simulink model "Fault_Tolerant_Motor_Control"  (R2023b)
settings: Solver=ode23  StartTime=0.0  StopTime=1  RelTol=1e-7
values from neighbouring files (symbols this model uses):
  a = 0.01    [Parameters.m]
  Fc_EMF = 60    [Parameters.m]
  Imax = 95    [Parameters.m]
  J = 0.01    [Parameters.m]
  K_SMO = 20    [Parameters.m]
  Kb_PLL = 50    [Parameters.m]
  Ki_PLL = 9    [Parameters.m]
  Ki_w = 210    [Parameters.m]
  Kp_PLL = 1    [Parameters.m]
  Kp_w = 2.9    [Parameters.m]
  Ld = 0.00047    [Parameters.m]
  Lq = 0.00047    [Parameters.m]
  m = 0.06    [Parameters.m]
  P = 4    [Parameters.m]
  Pmax = 50000    [Parameters.m]
  Psi = 0.1    [Parameters.m]
  Rs = 0.079    [Parameters.m]
  Te_max = 80    [Parameters.m]
  theta_offset = 0    [Parameters.m]
  Ts = 2e-6    (= 2e-06)    [Parameters.m]
  Tsc = 5e-05    [Parameters.m]
  Vdc = 370    [Parameters.m]
undefined symbols (not defined in the file or in its folder): DiscIntNeverNeededParam, ee_sli_rtmsupport, gcbh
libraries: fl_lib x18, nesl_utility x17, ee_lib x11, simulink x6, eeTransforms x2, mcbcontrolslib x2, eePmsmCurrentController x1, eePwmGeneratorTwoLevel x1, slpidlib x1, eeDiscretePi x1, batteryecm_lib x1, eeResolverToDigitalConverter x1
(part 1 of 2)
settings Model: Creator=sm103  LastModifiedBy=sm103
settings DebuggingCC: ParameterPrecisionLossMsg=none  UnderSpecifiedDimensionMsg=warning

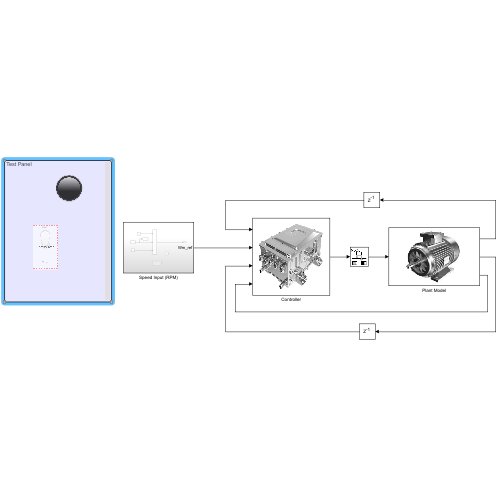
[thumbnail: Simulink's stored preview of the top-level diagram]
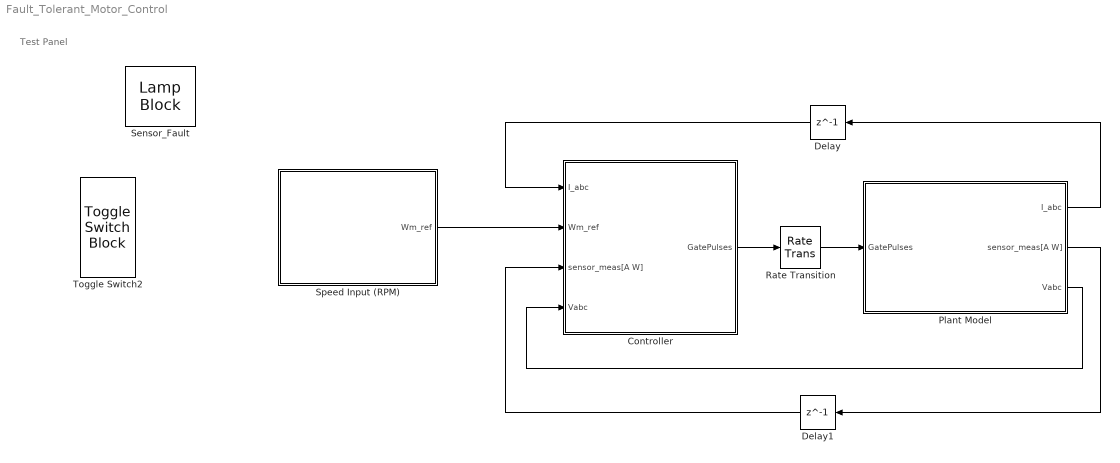
== system Fault_Tolerant_Motor_Control ==
  note: Test Panel
  Controller : Subsystem
      mask Display: image('ev-controller-4.jpeg');
  Delay : Delay  DelayLength=1
  Delay1 : Delay  DelayLength=1
  Plant Model : Subsystem
      mask Display: image('PMSM.jfif');
  Rate Transition : RateTransition  OutPortSampleTime=Ts
  Sensor_Fault : LampBlock  LabelPosition=Hide
  Speed Input (RPM) : Subsystem
  Toggle Switch2 : ToggleSwitchBlock  LabelPosition=Hide
      settings: Values={{'Stop', 'Start'}, [0 1]}
  wires:
  Controller/1(GatePulses) -> Rate Transition/1
  Rate Transition/1 -> Plant Model/1(GatePulses)
  Plant Model/1(I_abc) -> Delay/1
  Delay/1 -> Controller/1(I_abc)
  Plant Model/2(sensor_meas[A W]) -> Delay1/1
  Plant Model/3(Vabc) -> Controller/4(Vabc)
  Delay1/1 -> Controller/3(sensor_meas[A W])
  Speed Input (RPM)/1(Wm_ref) -> Controller/2(Wm_ref)

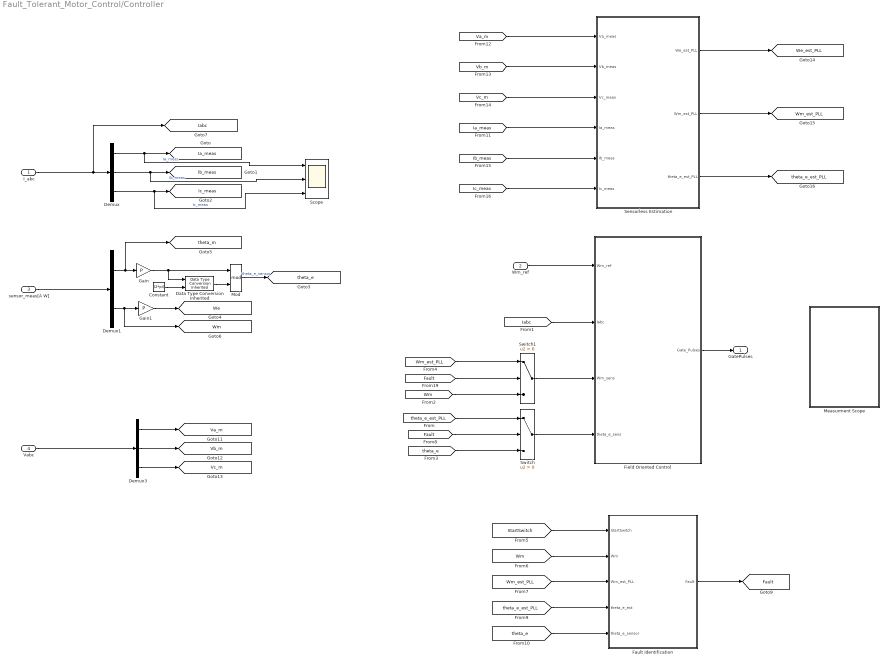
== system Fault_Tolerant_Motor_Control/Controller ==
  I_abc : Inport
  Wm_ref : Inport  Port=2
  sensor_meas[A W] : Inport  Port=3
  Vabc : Inport  Port=4
  Constant : Constant  Value=(2*pi)
  Data Type Conversion Inherited : simulink/Signal Attributes/Data Type Conversion Inherited  ConvertRealWorld=Real World Value  DoSatur=off
  Demux : Demux  Outputs=3
  Demux1 : Demux  Outputs=2
  Demux3 : Demux  Outputs=3
  Fault Identification : Subsystem
  Field Oriented Control : Subsystem
  Gain : Gain  Gain=P
  Gain1 : Gain  Gain=P
  Measurment Scope : Subsystem
  Mod : Math  Operator=mod
  Scope : Scope  NumInputPorts=3
  Sensorless Estimation : Subsystem
  Switch : Switch  Criteria=u2 > Threshold  SaturateOnIntegerOverflow=off  InputSameDT=off
  Switch1 : Switch  Criteria=u2 > Threshold  SaturateOnIntegerOverflow=off  InputSameDT=off
  GatePulses : Outport
  tag scope: Fault=global, Ia_meas=global, Iabc=global, Ib_meas=global, Ic_meas=global, Va_m=global, Vb_m=global, Vc_m=global, We=global, We_est_PLL=global, Wm=global, Wm_est_PLL=global, theta_e=global, theta_e_est_PLL=global, theta_m=global
  wires:
  I_abc/1 -> [Iabc], Demux/1
  Demux/1 -> Scope/1, [Ia_meas]  "Ia_meas"
  Demux/2 -> Scope/2, [Ib_meas]  "Ib_meas"
  Demux/3 -> Scope/3, [Ic_meas]  "Ic_meas"
  sensor_meas[A W]/1 -> Demux1/1
  Demux1/2 -> [Wm], Gain1/1
  Demux1/1 -> [theta_m], Gain/1
  Gain1/1 -> [We]
  Gain/1 -> Data Type Conversion Inherited/1, Mod/1
  Mod/1 -> [theta_e]  "theta_e_sensor"
  Data Type Conversion Inherited/1 -> Mod/2
  Constant/1 -> Data Type Conversion Inherited/2
  Vabc/1 -> Demux3/1
  Demux3/1 -> [Va_m]
  Demux3/2 -> [Vb_m]
  Demux3/3 -> [Vc_m]
  [Iabc] -> Field Oriented Control/2(Iabc)
  Field Oriented Control/1(Gate_Pulses) -> GatePulses/1
  Switch/1 -> Field Oriented Control/4(theta_e_sens)
  [theta_e_est_PLL] -> Switch/1
  Sensorless Estimation/1(We_est_PLL) -> [We_est_PLL]
  Sensorless Estimation/2(Wm_est_PLL) -> [Wm_est_PLL]
  Sensorless Estimation/3("theta_e_est_PLL ") -> [theta_e_est_PLL]
  [Va_m] -> Sensorless Estimation/1(Va_meas)
  [Vb_m] -> Sensorless Estimation/2(Vb_meas)
  [Vc_m] -> Sensorless Estimation/3(Vc_meas)
  Wm_ref/1 -> Field Oriented Control/1(Wm_ref)
  Fault Identification/1(Fault) -> [Fault]
  [StartSwitch] -> Fault Identification/1(StartSwitch)
  [Wm] -> Fault Identification/2(Wm)
  [Wm_est_PLL] -> Fault Identification/3(Wm_est_PLL)
  [theta_e_est_PLL] -> Fault Identification/4(theta_e_est)
  [theta_e] -> Fault Identification/5(theta_e_sensor)
  [Wm_est_PLL] -> Switch1/1
  [Wm] -> Switch1/3
  [Ia_meas] -> Sensorless Estimation/4(Ia_meas)
  [Ib_meas] -> Sensorless Estimation/5(Ib_meas)
  [Ic_meas] -> Sensorless Estimation/6(Ic_meas)
  [theta_e] -> Switch/3
  Switch1/1 -> Field Oriented Control/3(Wm_sens)
  [Fault] -> Switch/2
  [Fault] -> Switch1/2

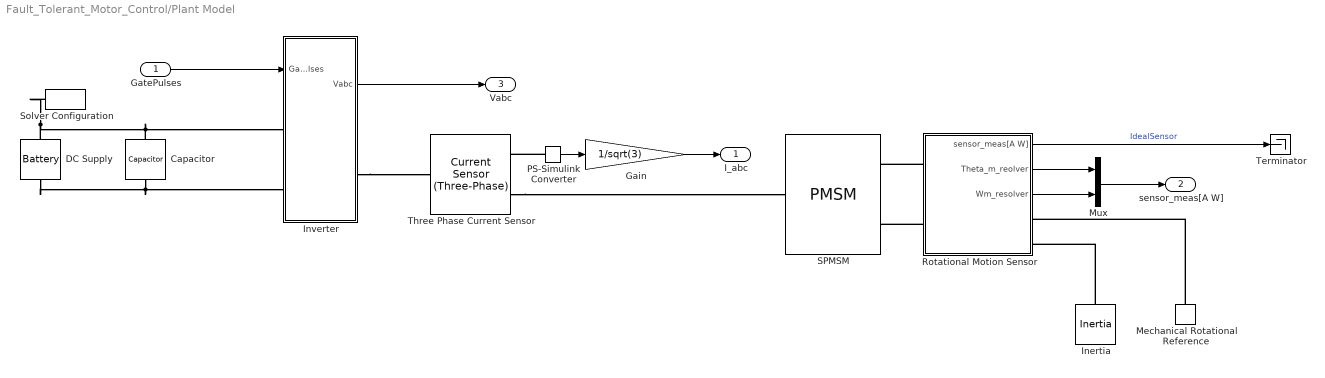
== system Fault_Tolerant_Motor_Control/Plant Model ==
  GatePulses : Inport
  Capacitor : ee_lib/Passive/Capacitor  cap_option=ee.enum.passive.capacitor.capOption.const  c=1e-6 F  Cvec=[1e-05, 1e-06] F  Vvec=[0, 10] V  CV_table_symmetry=ee.enum.passive.capacitor.tableSymmetry.yes  f_vec=[1, 10] kHz  DFext_vec=[.8, 1.2]  enable_C_tol=ee.enum.toleranceApplication.none  averaging_period=0 s  C_tol=5  tol_distribution=ee.enum.toleranceDistribution.uniform  nSigma=4  r=1e-6 Ohm  g=0 1/Ohm  enable_operating_limits=ee.enum.enable.no  operating_limit_action=ee.enum.passive.reportOpLim.warn  max_working_voltage_range=[-25, 25] V  power_rating=1 W  enable_faults=ee.enum.enable.no  fault_action=simscape.enum.assert.action.none  Cscale_faulted=100  R_faulted=1e-3 Ohm  G_faulted=0 1/Ohm  tau_fault=1e-3 s  fault_trigger=ee.enum.faults.faultTrigger.temporal  t_fault=1 s  max_permissible_voltage_range=[-100, 100] V  t_fail_on_voltage=1 s  i_specify=off  i_priority=None  i=0 A  i_nominal_specify=off  i_nominal_unit=A  i_nominal_value=1  v_specify=off  v_priority=None  v=0 V  v_nominal_specify=off  v_nominal_unit=V  v_nominal_value=1  vc_specify=off  vc_priority=High  vc=0 V  vc_nominal_specify=off  vc_nominal_unit=V  vc_nominal_value=1
  DC Supply : batteryecm_lib/Battery  Vnom=Vdc V  prm_dir=simscape.enum.battery.prm_dir.disabled  R1_dis=2 Ohm  R1_ch=2 Ohm  R1=0.01 Ohm  prm_AH=simscape.enum.battery.prm_AH.infinite  AH=50 A*hr  V1=11.5 V  AH1=25 A*hr  prm_R2=simscape.enum.battery.prm_R2.disabled  R2=2000 Ohm  Tmeas=298.15 K  charge_measurement_port=simscape.enum.battery.enable.no  prm_dyn=simscape.enum.battery.prm_dyn.off  Rp1=0.005 Ohm  tau1=30 s  Rp2=0.005 Ohm  tau2=30 s  Rp3=0.005 Ohm  tau3=30 s  Rp4=0.005 Ohm  tau4=30 s  Rp5=0.005 Ohm  tau5=30 s  prm_fade=simscape.enum.battery.prm_fade.disabled  N_fade=100  AH_fade=45 A*hr  R1_fade=2.02 Ohm  R1_ch_fade=2.02 Ohm  V1_fade=10.35 V  prm_age=simscape.enum.battery.prm_age.disabled  prm_age_OCV=simscape.enum.battery.prm_age_OCV.OCV  OCV_age=0.9  SOC_age=60  Tmeas_age=298.15 K  delta_time_age_vec=[0] d  temperature_age_vec=[273] K  OCV_scaling_age=2.2134e6  OCV_offset_age=1.632e6  temp_exp_age=0.515833569 V  t_exp_age=0.75  Vnom_T2=12 V  R1_T2=2.2 Ohm  R1_T2_dis=2.2 Ohm  R1_T2_ch=2.2 Ohm  V1_T2=11.4 V  R2_T2=2200 Ohm  Rp1_T2=0.005 Ohm  tau1_T2=30 s  Rp2_T2=0.005 Ohm  tau2_T2=30 s  Rp3_T2=0.005 Ohm  tau3_T2=30 s  Rp4_T2=0.005 Ohm  tau4_T2=30 s  Rp5_T2=0.005 Ohm  tau5_T2=30 s  Tmeas2=273.15 K  thermal_port=simscape.enum.thermaleffects.omit  thermal_mass=30000 J/K  i_specify=off  i_priority=None  i=0 A  i_nominal_specify=off  i_nominal_unit=A  i_nominal_value=1  v_specify=off  v_priority=None  v=0 V  v_nominal_specify=off  v_nominal_unit=V  v_nominal_value=1  charge_specify=on  charge_priority=High  charge=7000 A*hr  charge_nominal_specify=off  charge_nominal_unit=A*hr  charge_nominal_value=1  num_cycles_specify=off  num_cycles_priority=High  num_cycles=0  num_cycles_nominal_specify=off  num_cycles_nominal_unit=1  num_cycles_nominal_value=1  temperature_specify=off  temperature_priority=High  temperature=298.15 K  temperature_nominal_specify=off  temperature_nominal_unit=K  temperature_nominal_value=1
  Gain : Gain  Gain=1/sqrt(3)
  Inertia : fl_lib/Mechanical/Rotational Elements/Inertia  inertia=J kg*m^2  num_ports=foundation.enum.numPorts2.one  w_specify=on  w_priority=High  w=0 rad/s  w_nominal_specify=off  w_nominal_unit=rad/s  w_nominal_value=0  t_specify=off  t_priority=None  t=0 N*m  t_nominal_specify=off  t_nominal_unit=N*m  t_nominal_value=0
  Inverter : Subsystem
  Mechanical Rotational Reference : fl_lib/Mechanical/Rotational Elements/Mechanical Rotational Reference
  Mux : Mux  Inputs=2
  PS-Simulink Converter : nesl_utility/PS-Simulink Converter  PhysicalDomain=network_engine_domain  SubClassName=ps_output  LeftPortType=input  RightPortType=output  PseudoPeriodic=off  Frequencies=[]  VectorFormat=inherit  Unit=inherit  AffineConversion=off
  Rotational Motion Sensor : Subsystem
  SPMSM : ee_lib/Electromechanical/Permanent Magnet/PMSM  port_option=ee.enum.threePhasePort.composite  winding_type=ee.enum.statorconnection.wye  machine_param=ee.enum.pmsm.parameterization.constant  nPolePairs=P  pmflux_param=ee.enum.pmflux.fluxlinkage  pm_flux_linkage=Psi Wb  torque_constant=0.18 N*m/A  back_emf_constant=0.18 V*s/rad  stator_param=ee.enum.statorparam.LdLqL0  Ld=Ld H  Lq=Lq H  idVec=[-200, 0, 200] A  iqVec=[-200, 0, 200] A  LdMatrix=0.0002 * ones(3, 3) H  LqMatrix=0.0002 * ones(3, 3) H  PmMatrix=0.1 * ones(3, 3) Wb  ktMatrix=0.18 * ones(3, 3) N*m/A  keMatrix=0.18 * ones(3, 3) V*s/rad  L0=0.00016 H  Ls=0.0002 H  Lm=-0.00002 H  Ms=0.00002 H  Rs=Rs Ohm  zero_sequence=ee.enum.park.zerosequence.exclude  axes_param=ee.enum.rotorangle.qaxis  loss_param=ee.enum.ironloss.none  losses_oc=[0, 0, 0] W  losses_sc=[0, 0, 0] W  f_losses=60 Hz  Isc_losses=95 A  J=0.01 kg*m^2  lam=0 N*m*s/rad  i_d_specify=off  i_d_priority=None  i_d=0 A  i_d_nominal_specify=off  i_d_nominal_unit=A  i_d_nominal_value=1  i_q_specify=off  i_q_priority=None  i_q=0 A  i_q_nominal_specify=off  i_q_nominal_unit=A  i_q_nominal_value=1  torque_specify=off  torque_priority=None  torque=0 N*m  torque_nominal_specify=off  torque_nominal_unit=N*m  torque_nominal_value=1  angular_velocity_specify=on  angular_velocity_priority=High  angular_velocity=0 rpm  angular_velocity_nominal_specify=off  angular_velocity_nominal_unit=rpm  angular_velocity_nominal_value=1  angular_position_specify=on  angular_position_priority=High  angular_position=0 deg  angular_position_nominal_specify=off  angular_position_nominal_unit=deg  angular_position_nominal_value=1  alpha=3.93e-3 1/K  alpha_flux=-0.001 1/K  Tmeas=298.15 K  stator_thermal_mass=100 J/K  rotor_thermal_mass=200 J/K  Rm_percent_rotor=90  Rd_percent_rotor=30  temperatureA_specify=off  temperatureA_priority=High  temperatureA=25 degC  temperatureA_nominal_specify=off  temperatureA_nominal_unit=degC  temperatureA_nominal_value=1  temperatureB_specify=off  temperatureB_priority=High  temperatureB=25 degC  temperatureB_nominal_specify=off  temperatureB_nominal_unit=degC  temperatureB_nominal_value=1  temperatureC_specify=off  temperatureC_priority=High  temperatureC=25 degC  temperatureC_nominal_specify=off  temperatureC_nominal_unit=degC  temperatureC_nominal_value=1  temperatureR_specify=off  temperatureR_priority=High  temperatureR=25 degC  temperatureR_nominal_specify=off  temperatureR_nominal_unit=degC  temperatureR_nominal_value=1
      settings: InternalSimscapePortConfiguration="{\"Bottom\":[],\"Left\":[{\"id\":\"N\",\"label\":\"~\",\"type\":\"foundation.electrical.three_phase\"}],\"Right\":[{\"id\":\"R\",\"label\":\"R\",\"type\":\"foundation.mechanical.rotational.rotational\"},{\"id\":\"C\",\"label\":\"C\",\"type\":\"foundation.mechanical.rotational.rotational\"}],\"Top\":[]}"
  Solver Configuration : nesl_utility/Solver Configuration  PhysicalDomain=network_engine_domain  SubClassName=solver  LeftPortType=input  RightPortType=generic  Tones=[]  Harmonics=[]  SimulateNoise=off  Profile=off  UseLocalSampling=off  EnableSwitchedLinearOptims=on  FrequencyDomain=off  UseCCode=off  RelTol=0.001  AbsTol=1e-06  MinStep=1e-09  ToWorkspace=off  RevertToSquareIcSolve=off  NumHomotopyIterations=100  PhasorMode=off  PhasorModeNumHarmonics=1  ConsistencySolver=NEWTON_FTOL  IndexReductionMethod=DerivativeReplacement  DoDC=off  ResidualTolerance=1e-9  ConsistencyTolSource=GLOBAL  ConsistencyAbsTol=0.001  ConsistencyRelTol=0.001  ConsistencyTolFactor=0.001  UseLocalSolver=on  LocalSolverChoice=NE_BACKWARD_EULER_ADVANCER  ResolveIndetEquations=on  FunctionEvalNumThread=1  LocalSolverSampleTime=Ts  DoFixedCost=on  MaxNonlinIter=4  MaxModeIter=2  ComputeImpulses=off  ImpulseIterations=2  LinearAlgebra=auto  LinearAlgebraNumThread=0  EquationFormulation=NE_TIME_EF  DelaysMemoryBudget=1024  AutomaticFiltering=on  FilteringTimeConstant=0.001  PartitionStorageMethod=AS_NEEDED  PartitionMemoryBudget=1024  PartitionMethod=FAST  MultibodyUseLocalSolver=off  MultibodyLocalSolverChoice=ODE1  MultibodyLocalSolverSampleTime=0.001
  Terminator : Terminator
  Three Phase Current Sensor : ee_lib/Sensors & Transducers/Current Sensor (Three-Phase)
  I_abc : Outport
  sensor_meas[A W] : Outport  Port=2
  Vabc : Outport  Port=3
  wires:
  Gain/1 -> I_abc/1
  PS-Simulink Converter/1 -> Gain/1
  Rotational Motion Sensor/1(sensor_meas[A W]) -> Terminator/1  "IdealSensor"
  GatePulses/1 -> Inverter/1(GatePulses)
  Inverter/1(Vabc) -> Vabc/1
  Rotational Motion Sensor/2(Theta_m_reolver) -> Mux/1
  Rotational Motion Sensor/3(Wm_resolver) -> Mux/2
  Mux/1 -> sensor_meas[A W]/1
  connections:
  Three Phase Current Sensor/RConn2 -- SPMSM/LConn1
  Mechanical Rotational Reference/LConn1 -- Rotational Motion Sensor/RConn1
  DC Supply/LConn1 -- Inverter/LConn1 -- Capacitor/LConn1 -- Solver Configuration/RConn1
  Inverter/RConn1 -- Three Phase Current Sensor/LConn1
  PS-Simulink Converter/LConn1 -- Three Phase Current Sensor/RConn1
  Rotational Motion Sensor/LConn1 -- SPMSM/RConn1
  DC Supply/RConn1 -- Capacitor/RConn1 -- Inverter/LConn2
  Rotational Motion Sensor/LConn2 -- SPMSM/RConn2
  Inertia/LConn1 -- Rotational Motion Sensor/RConn2

== system Fault_Tolerant_Motor_Control/Speed Input (RPM) ==
  Constant : Constant  Commented=on  Value=1000
  Constant2 : Constant
  Constant3 : Constant  Value=0
  Signal Editor : SignalEditorBlockLib/Signal Editor  Commented=on  FileName=SpeedProfile1.mat  ActiveScenario=Scenario  ActiveSignal=Signal 1  IsBus=off  OutputBusObjectStr=Bus: BusObject  SampleTime=0  Interpolate=off  ZeroCross=off  OutputAfterFinalValue=Setting to zero  Unit=inherit  PreserveSignalName=on  ApplySigPropsToAllScenarios=on  ApplySigPropsToAllSignals=off
  Step : Step  Time=0.5  Before=1000  After=2000  SampleTime=0
  Switch1 : Switch  Criteria=u2 > Threshold  SaturateOnIntegerOverflow=off  InputSameDT=off
  Wm_ref : Outport
  tag scope: StartSwitch=global
  wires:
  Constant2/1 -> [StartSwitch], Switch1/2
  Constant3/1 -> Switch1/3
  Step/1 -> Switch1/1
  Switch1/1 -> Wm_ref/1

== system Fault_Tolerant_Motor_Control/Controller/Fault Identification ==
  StartSwitch : Inport
  Wm : Inport  Port=2
  Wm_est_PLL : Inport  Port=3
  theta_e_est : Inport  Port=4
  theta_e_sensor : Inport  Port=5
  Chart : Stateflow chart  TreatAsAtomicUnit=on
  Fault : Outport
  wires:
  Wm/1 -> Chart/2(Wm)
  StartSwitch/1 -> Chart/1(StartSwitch)
  Wm_est_PLL/1 -> Chart/3(Wm_est_PLL)
  Chart/1(Fault) -> Fault/1
  theta_e_est/1 -> Chart/4(theta_e_est)
  theta_e_sensor/1 -> Chart/5(theta_e_sensor)

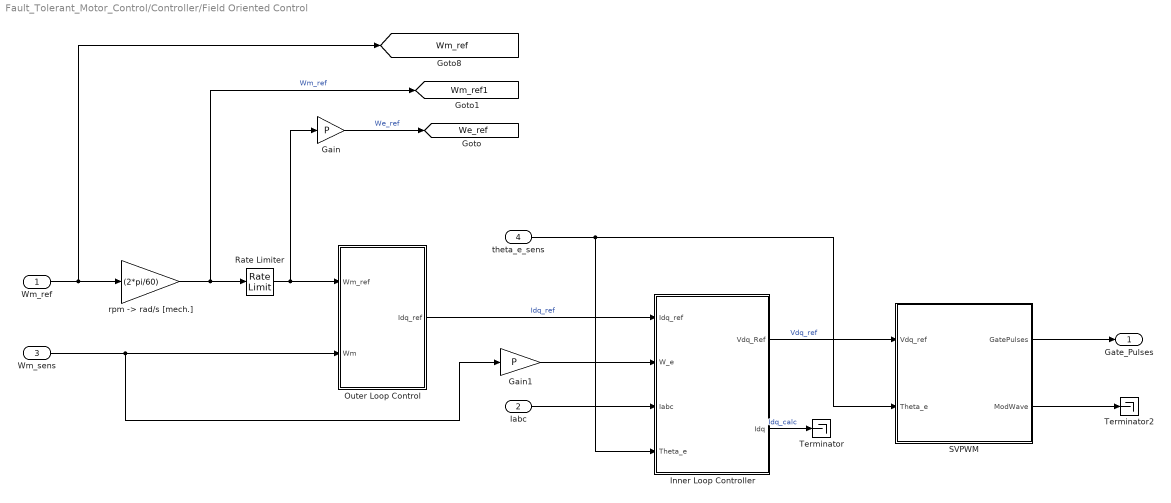
== system Fault_Tolerant_Motor_Control/Controller/Field Oriented Control ==
  Wm_ref : Inport
  Iabc : Inport  Port=2
  Wm_sens : Inport  Port=3
  theta_e_sens : Inport  Port=4
  Gain : Gain  Gain=P
  Gain1 : Gain  Gain=P
  Inner Loop Controller : Subsystem
  Outer Loop Control : Subsystem
  Rate Limiter : RateLimiter  RisingSlewLimit=(Te_max/J)  FallingSlewLimit=-(Te_max/J)  SampleTimeMode=inherited
  SVPWM : Subsystem
  Terminator : Terminator
  Terminator2 : Terminator
  "rpm -> rad/s [mech.]" : Gain  Gain=(2*pi/60)
  Gate_Pulses : Outport
  tag scope: We_ref=global, Wm_ref1=global, Wm_ref=global
  wires:
  Wm_ref/1 -> "rpm -> rad/s [mech.]"/1, [Wm_ref]
  "rpm -> rad/s [mech.]"/1 -> [Wm_ref1], Rate Limiter/1  "Wm_ref"
  Rate Limiter/1 -> Gain/1, Outer Loop Control/1(Wm_ref)
  Iabc/1 -> Inner Loop Controller/3(Iabc)
  Wm_sens/1 -> Outer Loop Control/2(Wm), Gain1/1
  theta_e_sens/1 -> Inner Loop Controller/4(Theta_e), SVPWM/2(Theta_e)
  Gain/1 -> [We_ref]  "We_ref"
  Outer Loop Control/1(Idq_ref) -> Inner Loop Controller/1(Idq_ref)  "Idq_ref"
  Inner Loop Controller/1(Vdq_Ref) -> SVPWM/1(Vdq_ref)  "Vdq_ref"
  Gain1/1 -> Inner Loop Controller/2(W_e)
  SVPWM/1(GatePulses) -> Gate_Pulses/1
  Inner Loop Controller/2(Idq) -> Terminator/1  "Idq_calc"
  SVPWM/2(ModWave) -> Terminator2/1

== system Fault_Tolerant_Motor_Control/Controller/Measurment Scope ==
  Position Error : Subsystem
  Scope : Scope  NumInputPorts=10
  Speed Error : Subsystem
  wires:
  [theta_e] -> Scope/4  "Resolver Electrical Angle (rad)"
  [theta_e_est_PLL] -> Scope/5  "Estimated Electrical Angle (rad)"
  [Wm_est_PLL] -> Scope/2  "Estimated Mechanical Speed (rad/s)"
  [Wm] -> Scope/3  "Resolver Mechanical Speed (rad/s)"
  [Wm_ref1] -> Scope/1  "Mechanical Speed Reference (rad/s)"
  Speed Error/1(Out1) -> Scope/6  "Speed Error (rad/s)"
  Position Error/1(Out1) -> Scope/7  "Position Error (rad)"
  [Fault] -> Scope/8  "Sensor Fault"
  [theta_e_testSensor] -> Scope/9  "Electrical angle test sensor (rad)"
  [Wm_testSensor] -> Scope/10  "Mechanical Speed from test sensor (rad/s)"

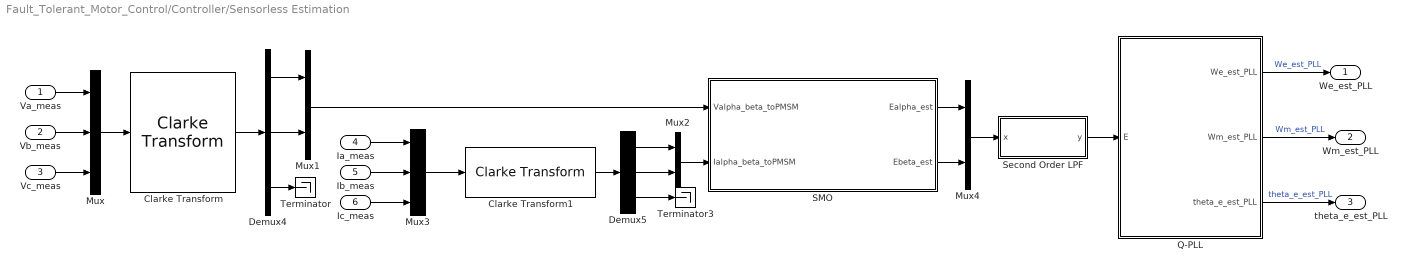
== system Fault_Tolerant_Motor_Control/Controller/Sensorless Estimation ==
  Va_meas : Inport
  Vb_meas : Inport  Port=2
  Vc_meas : Inport  Port=3
  Ia_meas : Inport  Port=4
  Ib_meas : Inport  Port=5
  Ic_meas : Inport  Port=6
  Clarke Transform : mcbcontrolslib/Clarke Transform  VariantControl=Variant2  PhaseInput=Three inputs  EnPowerInv=off
      settings: LibrarySourceBlock=mcbhdllib/Controls/Math Transforms/Clarke Transform
  Clarke Transform1 : mcbcontrolslib/Clarke Transform  VariantControl=Variant2  PhaseInput=Three inputs  EnPowerInv=off
      settings: LibrarySourceBlock=mcbhdllib/Controls/Math Transforms/Clarke Transform
  Demux4 : Demux  Outputs=3
  Demux5 : Demux  Outputs=3
  Mux : Mux  Inputs=3
  Mux1 : Mux  Inputs=2
  Mux2 : Mux  Inputs=2
  Mux3 : Mux  Inputs=3
  Mux4 : Mux  Inputs=2
  Q-PLL : Subsystem
  SMO : Subsystem
  Second Order LPF : Subsystem
  Terminator : Terminator
  Terminator3 : Terminator
  We_est_PLL : Outport
  Wm_est_PLL : Outport  Port=2
  "theta_e_est_PLL " : Outport  Port=3
  wires:
  Demux4/2 -> Mux1/2
  Q-PLL/2(Wm_est_PLL) -> Wm_est_PLL/1  "Wm_est_PLL"
  Demux5/3 -> Terminator3/1
  Mux2/1 -> SMO/2(Ialpha_beta_toPMSM)
  Mux3/1 -> Clarke Transform1/1
  Demux5/2 -> Mux2/2
  Demux5/1 -> Mux2/1
  Va_meas/1 -> Mux/1
  Mux/1 -> Clarke Transform/1
  Vb_meas/1 -> Mux/2
  Demux4/3 -> Terminator/1
  Clarke Transform/1 -> Demux4/1
  Q-PLL/1(We_est_PLL) -> We_est_PLL/1  "We_est_PLL"
  Ic_meas/1 -> Mux3/3
  Ia_meas/1 -> Mux3/1
  Mux1/1 -> SMO/1(Valpha_beta_toPMSM)
  Clarke Transform1/1 -> Demux5/1
  Ib_meas/1 -> Mux3/2
  Vc_meas/1 -> Mux/3
  Demux4/1 -> Mux1/1
  Q-PLL/3(theta_e_est_PLL) -> "theta_e_est_PLL "/1  "theta_e_est_PLL"
  SMO/1(Ealpha_est) -> Mux4/1
  SMO/2(Ebeta_est) -> Mux4/2
  Second Order LPF/1(y) -> Q-PLL/1(E)
  Mux4/1 -> Second Order LPF/1(x)

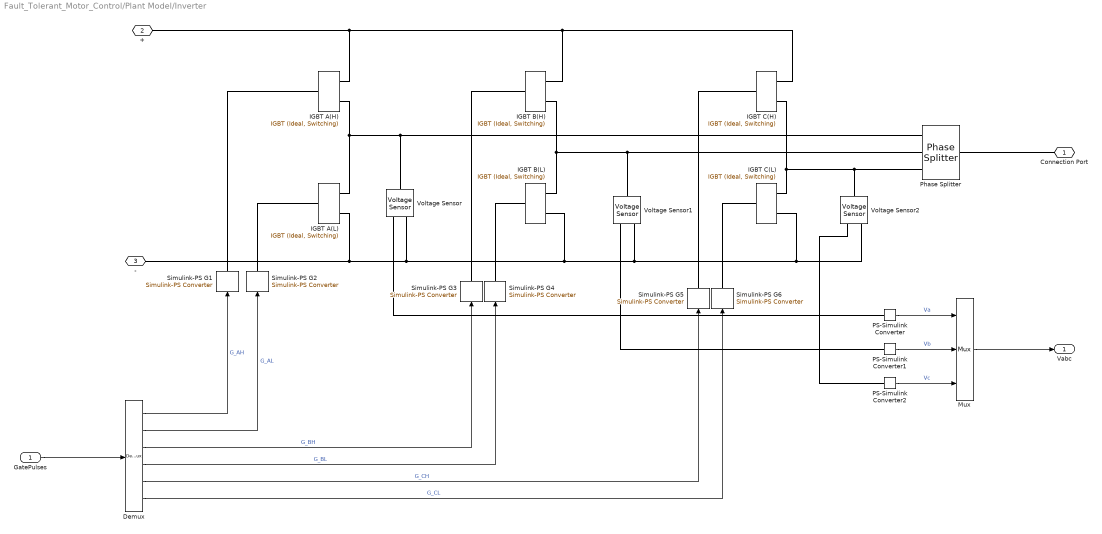
== system Fault_Tolerant_Motor_Control/Plant Model/Inverter ==
  GatePulses : Inport
  Demux : Demux  Outputs=6
  IGBT A(H) : ee_lib/Semiconductors & Converters/IGBT (Ideal, Switching)  port_option=ee.enum.controlport.ps  Vf=0.8 V  Ron=0.001 Ohm  Goff=1e-5 S  Vth=0.5 V  diode_param=ee.enum.converters.protectiondiode.nodynamics  diode_Vf=0.8 V  diode_Ron=0.001 Ohm  diode_Goff=1e-5 S  diode_C=5e-8 F  diode_iRM=-235 A  diode_iF=300 A  diode_idot=-50 A/us  diode_trr_param=1  diode_trr_factor=3  diode_trr=15 us  diode_Qrr=1.5e+3 s*uA  ice_specify=off  ice_priority=None  ice=0 A  ice_nominal_specify=off  ice_nominal_unit=A  ice_nominal_value=1  vce_specify=off  vce_priority=None  vce=0 V  vce_nominal_specify=off  vce_nominal_unit=V  vce_nominal_value=1  vge_specify=off  vge_priority=None  vge=0 V  vge_nominal_specify=off  vge_nominal_unit=V  vge_nominal_value=1  thermal_loss_option=ee.enum.converters.thermalLossOption.constantvalues  Von_data=[0, .1, .6, .8, 1, 1.3, 1.6, 2, 2.4; 0, .1, .7, 1, 1.2, 1.5, 1.9, 2.4, 2.8] V  Tj=[298.15, 398.15] K  Iout_data=[0, .1, 1, 5, 10, 20, 40, 70, 100] A  Eon_data=[0, .0024, .024, .12, .2, .48, 1.04, 2.16, 3.24; 0, .003, .03, .15, .25, .6, 1.3, 2.7, 4.05] * 1e-3 J  Eoff_data=[0, .0007, .0066, .033, .066, .17, .33, .83, 1.5; 0, .001, .01, .05, .1, .25, .5, 1.2, 2.2] * 1e-3 J  Eon_data_3D=[zeros(2, 9, 3)] J  Eoff_data_3D=[zeros(2, 9, 3)] J  Tj_loss=[298.15, 398.15] K  Iout_data_loss=[0, .1, 1, 5, 10, 20, 40, 70, 100] A  tabulateWithVce=false  Vce_loss=[0, 150, 300] V  Eon_scalar=22.86e-3 J  Eoff_scalar=17.14e-3 J  Voff=300 V  Iout_scalar=600 A  useCurrentFromPreviousCycle=false  useVoltageFromPreviousCycle=false  diodeModelType=ee.enum.converters.diodeModelType.pwl  diodeTableType=ee.enum.diode.tableType.IfMat  diode_IfMat=[.07, .12, .19, 1.75, 4.24, 7.32, 11.2; .16, .3, .72, 2.14, 4.02, 6.35, 9.12] A  diode_VfMat=[.9, 1.15, 1.25, 1.5, 1.75, 2.17, 2.6, 2.85; .58, .68, .75, 1.1, 1.38, 1.77, 2.27, 2.7] V  diode_TjVec=[25, 125] degC  diode_VfVec=[.5, .7, .9, 1.3, 1.7, 2.1, 2.5] V  diode_IfVec=[.1, .2, .5, 1, 2, 4, 7, 10] A  diode_Vr=-600 V  diode_Ls=150 nH  diode_Erec=0.03 J  diode_rec_loss_model=ee.enum.diode.reverseRecoveryModel.fixed  diode_ErecVal=0 J  diode_scaleWithIandV=true  diode_ErecMat=zeros(2, 3) J  diode_TjrecVec=[298.15, 398.15] K  diode_IfrecVec=[.1, 1, 10] A  diode_IrecVal=10 A  diode_VrecVal=10 V  diode_tFilter=1 / 1000 / 100 s  thermal_network_parameterization=ee.enum.thermalNetworkTopology.external  Rth=[.08, .5] K/W  Rth_Cauer=[.08, .1, .5] K/W  Rth_Foster=[.08, .14, .22, .16] K/W  thermal_mass_parameterization=ee.enum.thermalNetwork.timeconstant  thermal_mass=[.01, .5] J/K  thermal_mass_Cauer=[.01, .1, .5] J/K  thermal_mass_Foster=[.001, .005, .05, .5] J/K  thermal_time_constant=[.001, .2] s  thermal_time_constant_Cauer=[.001, .1, .2] s  thermal_time_constant_Foster=[7e-05, .0007, .01, .08] s  thermal_mass_initial_temperatures=[25, 25] degC  thermal_mass_initial_temperatures_Cauer=[25, 25, 25] degC  junction_thermal_mass=0.01 J/K  Tvec_initial_Foster=[25, 25, 25, 25] degC  no_thermal_network=0  junction_temperature_specify=off  junction_temperature_priority=None  junction_temperature=25 degC  junction_temperature_nominal_specify=off  junction_temperature_nominal_unit=degC  junction_temperature_nominal_value=1  Qj_specify=off  Qj_priority=None  Qj=0 W  Qj_nominal_specify=off  Qj_nominal_unit=W  Qj_nominal_value=1  accumulatedSwitchingLosses_specify=off  accumulatedSwitchingLosses_priority=None  accumulatedSwitchingLosses=0 J
  IGBT A(L) : ee_lib/Semiconductors & Converters/IGBT (Ideal, Switching)  port_option=ee.enum.controlport.ps  Vf=0.8 V  Ron=0.001 Ohm  Goff=1e-5 S  Vth=0.5 V  diode_param=2  diode_Vf=0.8 V  diode_Ron=0.001 Ohm  diode_Goff=1e-5 S  diode_C=5e-8 F  diode_iRM=-235 A  diode_iF=300 A  diode_idot=-50 A/us  diode_trr_param=1  diode_trr_factor=3  diode_trr=15 us  diode_Qrr=1.5e+3 s*uA  ice_specify=off  ice_priority=None  ice=0 A  ice_nominal_specify=off  ice_nominal_unit=A  ice_nominal_value=1  vce_specify=off  vce_priority=None  vce=0 V  vce_nominal_specify=off  vce_nominal_unit=V  vce_nominal_value=1  vge_specify=off  vge_priority=None  vge=0 V  vge_nominal_specify=off  vge_nominal_unit=V  vge_nominal_value=1  thermal_loss_option=ee.enum.converters.thermalLossOption.constantvalues  Von_data=[0, .1, .6, .8, 1, 1.3, 1.6, 2, 2.4; 0, .1, .7, 1, 1.2, 1.5, 1.9, 2.4, 2.8] V  Tj=[298.15, 398.15] K  Iout_data=[0, .1, 1, 5, 10, 20, 40, 70, 100] A  Eon_data=[0, .0024, .024, .12, .2, .48, 1.04, 2.16, 3.24; 0, .003, .03, .15, .25, .6, 1.3, 2.7, 4.05] * 1e-3 J  Eoff_data=[0, .0007, .0066, .033, .066, .17, .33, .83, 1.5; 0, .001, .01, .05, .1, .25, .5, 1.2, 2.2] * 1e-3 J  Eon_data_3D=[zeros(2, 9, 3)] J  Eoff_data_3D=[zeros(2, 9, 3)] J  Tj_loss=[298.15, 398.15] K  Iout_data_loss=[0, .1, 1, 5, 10, 20, 40, 70, 100] A  tabulateWithVce=false  Vce_loss=[0, 150, 300] V  Eon_scalar=22.86e-3 J  Eoff_scalar=17.14e-3 J  Voff=300 V  Iout_scalar=600 A  useCurrentFromPreviousCycle=false  useVoltageFromPreviousCycle=false  diodeModelType=ee.enum.converters.diodeModelType.pwl  diodeTableType=ee.enum.diode.tableType.IfMat  diode_IfMat=[.07, .12, .19, 1.75, 4.24, 7.32, 11.2; .16, .3, .72, 2.14, 4.02, 6.35, 9.12] A  diode_VfMat=[.9, 1.15, 1.25, 1.5, 1.75, 2.17, 2.6, 2.85; .58, .68, .75, 1.1, 1.38, 1.77, 2.27, 2.7] V  diode_TjVec=[25, 125] degC  diode_VfVec=[.5, .7, .9, 1.3, 1.7, 2.1, 2.5] V  diode_IfVec=[.1, .2, .5, 1, 2, 4, 7, 10] A  diode_Vr=-600 V  diode_Ls=150 nH  diode_Erec=0.03 J  diode_rec_loss_model=ee.enum.diode.reverseRecoveryModel.fixed  diode_ErecVal=0 J  diode_scaleWithIandV=true  diode_ErecMat=zeros(2, 3) J  diode_TjrecVec=[298.15, 398.15] K  diode_IfrecVec=[.1, 1, 10] A  diode_IrecVal=10 A  diode_VrecVal=10 V  diode_tFilter=1 / 1000 / 100 s  thermal_network_parameterization=ee.enum.thermalNetworkTopology.external  Rth=[.08, .5] K/W  Rth_Cauer=[.08, .1, .5] K/W  Rth_Foster=[.08, .14, .22, .16] K/W  thermal_mass_parameterization=ee.enum.thermalNetwork.timeconstant  thermal_mass=[.01, .5] J/K  thermal_mass_Cauer=[.01, .1, .5] J/K  thermal_mass_Foster=[.001, .005, .05, .5] J/K  thermal_time_constant=[.001, .2] s  thermal_time_constant_Cauer=[.001, .1, .2] s  thermal_time_constant_Foster=[7e-05, .0007, .01, .08] s  thermal_mass_initial_temperatures=[25, 25] degC  thermal_mass_initial_temperatures_Cauer=[25, 25, 25] degC  junction_thermal_mass=0.01 J/K  Tvec_initial_Foster=[25, 25, 25, 25] degC  no_thermal_network=0  junction_temperature_specify=off  junction_temperature_priority=None  junction_temperature=25 degC  junction_temperature_nominal_specify=off  junction_temperature_nominal_unit=degC  junction_temperature_nominal_value=1  Qj_specify=off  Qj_priority=None  Qj=0 W  Qj_nominal_specify=off  Qj_nominal_unit=W  Qj_nominal_value=1  accumulatedSwitchingLosses_specify=off  accumulatedSwitchingLosses_priority=None  accumulatedSwitchingLosses=0 J
  IGBT B(H) : ee_lib/Semiconductors & Converters/IGBT (Ideal, Switching)  port_option=ee.enum.controlport.ps  Vf=0.8 V  Ron=0.001 Ohm  Goff=1e-5 S  Vth=0.5 V  diode_param=2  diode_Vf=0.8 V  diode_Ron=0.001 Ohm  diode_Goff=1e-5 S  diode_C=5e-8 F  diode_iRM=-235 A  diode_iF=300 A  diode_idot=-50 A/us  diode_trr_param=1  diode_trr_factor=3  diode_trr=15 us  diode_Qrr=1.5e+3 s*uA  ice_specify=off  ice_priority=None  ice=0 A  ice_nominal_specify=off  ice_nominal_unit=A  ice_nominal_value=1  vce_specify=off  vce_priority=None  vce=0 V  vce_nominal_specify=off  vce_nominal_unit=V  vce_nominal_value=1  vge_specify=off  vge_priority=None  vge=0 V  vge_nominal_specify=off  vge_nominal_unit=V  vge_nominal_value=1  thermal_loss_option=ee.enum.converters.thermalLossOption.constantvalues  Von_data=[0, .1, .6, .8, 1, 1.3, 1.6, 2, 2.4; 0, .1, .7, 1, 1.2, 1.5, 1.9, 2.4, 2.8] V  Tj=[298.15, 398.15] K  Iout_data=[0, .1, 1, 5, 10, 20, 40, 70, 100] A  Eon_data=[0, .0024, .024, .12, .2, .48, 1.04, 2.16, 3.24; 0, .003, .03, .15, .25, .6, 1.3, 2.7, 4.05] * 1e-3 J  Eoff_data=[0, .0007, .0066, .033, .066, .17, .33, .83, 1.5; 0, .001, .01, .05, .1, .25, .5, 1.2, 2.2] * 1e-3 J  Eon_data_3D=[zeros(2, 9, 3)] J  Eoff_data_3D=[zeros(2, 9, 3)] J  Tj_loss=[298.15, 398.15] K  Iout_data_loss=[0, .1, 1, 5, 10, 20, 40, 70, 100] A  tabulateWithVce=false  Vce_loss=[0, 150, 300] V  Eon_scalar=22.86e-3 J  Eoff_scalar=17.14e-3 J  Voff=300 V  Iout_scalar=600 A  useCurrentFromPreviousCycle=false  useVoltageFromPreviousCycle=false  diodeModelType=ee.enum.converters.diodeModelType.pwl  diodeTableType=ee.enum.diode.tableType.IfMat  diode_IfMat=[.07, .12, .19, 1.75, 4.24, 7.32, 11.2; .16, .3, .72, 2.14, 4.02, 6.35, 9.12] A  diode_VfMat=[.9, 1.15, 1.25, 1.5, 1.75, 2.17, 2.6, 2.85; .58, .68, .75, 1.1, 1.38, 1.77, 2.27, 2.7] V  diode_TjVec=[25, 125] degC  diode_VfVec=[.5, .7, .9, 1.3, 1.7, 2.1, 2.5] V  diode_IfVec=[.1, .2, .5, 1, 2, 4, 7, 10] A  diode_Vr=-600 V  diode_Ls=150 nH  diode_Erec=0.03 J  diode_rec_loss_model=ee.enum.diode.reverseRecoveryModel.fixed  diode_ErecVal=0 J  diode_scaleWithIandV=true  diode_ErecMat=zeros(2, 3) J  diode_TjrecVec=[298.15, 398.15] K  diode_IfrecVec=[.1, 1, 10] A  diode_IrecVal=10 A  diode_VrecVal=10 V  diode_tFilter=1 / 1000 / 100 s  thermal_network_parameterization=ee.enum.thermalNetworkTopology.external  Rth=[.08, .5] K/W  Rth_Cauer=[.08, .1, .5] K/W  Rth_Foster=[.08, .14, .22, .16] K/W  thermal_mass_parameterization=ee.enum.thermalNetwork.timeconstant  thermal_mass=[.01, .5] J/K  thermal_mass_Cauer=[.01, .1, .5] J/K  thermal_mass_Foster=[.001, .005, .05, .5] J/K  thermal_time_constant=[.001, .2] s  thermal_time_constant_Cauer=[.001, .1, .2] s  thermal_time_constant_Foster=[7e-05, .0007, .01, .08] s  thermal_mass_initial_temperatures=[25, 25] degC  thermal_mass_initial_temperatures_Cauer=[25, 25, 25] degC  junction_thermal_mass=0.01 J/K  Tvec_initial_Foster=[25, 25, 25, 25] degC  no_thermal_network=0  junction_temperature_specify=off  junction_temperature_priority=None  junction_temperature=25 degC  junction_temperature_nominal_specify=off  junction_temperature_nominal_unit=degC  junction_temperature_nominal_value=1  Qj_specify=off  Qj_priority=None  Qj=0 W  Qj_nominal_specify=off  Qj_nominal_unit=W  Qj_nominal_value=1  accumulatedSwitchingLosses_specify=off  accumulatedSwitchingLosses_priority=None  accumulatedSwitchingLosses=0 J
  IGBT B(L) : ee_lib/Semiconductors & Converters/IGBT (Ideal, Switching)  port_option=ee.enum.controlport.ps  Vf=0.8 V  Ron=0.001 Ohm  Goff=1e-5 S  Vth=0.5 V  diode_param=2  diode_Vf=0.8 V  diode_Ron=0.001 Ohm  diode_Goff=1e-5 S  diode_C=5e-8 F  diode_iRM=-235 A  diode_iF=300 A  diode_idot=-50 A/us  diode_trr_param=1  diode_trr_factor=3  diode_trr=15 us  diode_Qrr=1.5e+3 s*uA  ice_specify=off  ice_priority=None  ice=0 A  ice_nominal_specify=off  ice_nominal_unit=A  ice_nominal_value=1  vce_specify=off  vce_priority=None  vce=0 V  vce_nominal_specify=off  vce_nominal_unit=V  vce_nominal_value=1  vge_specify=off  vge_priority=None  vge=0 V  vge_nominal_specify=off  vge_nominal_unit=V  vge_nominal_value=1  thermal_loss_option=ee.enum.converters.thermalLossOption.constantvalues  Von_data=[0, .1, .6, .8, 1, 1.3, 1.6, 2, 2.4; 0, .1, .7, 1, 1.2, 1.5, 1.9, 2.4, 2.8] V  Tj=[298.15, 398.15] K  Iout_data=[0, .1, 1, 5, 10, 20, 40, 70, 100] A  Eon_data=[0, .0024, .024, .12, .2, .48, 1.04, 2.16, 3.24; 0, .003, .03, .15, .25, .6, 1.3, 2.7, 4.05] * 1e-3 J  Eoff_data=[0, .0007, .0066, .033, .066, .17, .33, .83, 1.5; 0, .001, .01, .05, .1, .25, .5, 1.2, 2.2] * 1e-3 J  Eon_data_3D=[zeros(2, 9, 3)] J  Eoff_data_3D=[zeros(2, 9, 3)] J  Tj_loss=[298.15, 398.15] K  Iout_data_loss=[0, .1, 1, 5, 10, 20, 40, 70, 100] A  tabulateWithVce=false  Vce_loss=[0, 150, 300] V  Eon_scalar=22.86e-3 J  Eoff_scalar=17.14e-3 J  Voff=300 V  Iout_scalar=600 A  useCurrentFromPreviousCycle=false  useVoltageFromPreviousCycle=false  diodeModelType=ee.enum.converters.diodeModelType.pwl  diodeTableType=ee.enum.diode.tableType.IfMat  diode_IfMat=[.07, .12, .19, 1.75, 4.24, 7.32, 11.2; .16, .3, .72, 2.14, 4.02, 6.35, 9.12] A  diode_VfMat=[.9, 1.15, 1.25, 1.5, 1.75, 2.17, 2.6, 2.85; .58, .68, .75, 1.1, 1.38, 1.77, 2.27, 2.7] V  diode_TjVec=[25, 125] degC  diode_VfVec=[.5, .7, .9, 1.3, 1.7, 2.1, 2.5] V  diode_IfVec=[.1, .2, .5, 1, 2, 4, 7, 10] A  diode_Vr=-600 V  diode_Ls=150 nH  diode_Erec=0.03 J  diode_rec_loss_model=ee.enum.diode.reverseRecoveryModel.fixed  diode_ErecVal=0 J  diode_scaleWithIandV=true  diode_ErecMat=zeros(2, 3) J  diode_TjrecVec=[298.15, 398.15] K  diode_IfrecVec=[.1, 1, 10] A  diode_IrecVal=10 A  diode_VrecVal=10 V  diode_tFilter=1 / 1000 / 100 s  thermal_network_parameterization=ee.enum.thermalNetworkTopology.external  Rth=[.08, .5] K/W  Rth_Cauer=[.08, .1, .5] K/W  Rth_Foster=[.08, .14, .22, .16] K/W  thermal_mass_parameterization=ee.enum.thermalNetwork.timeconstant  thermal_mass=[.01, .5] J/K  thermal_mass_Cauer=[.01, .1, .5] J/K  thermal_mass_Foster=[.001, .005, .05, .5] J/K  thermal_time_constant=[.001, .2] s  thermal_time_constant_Cauer=[.001, .1, .2] s  thermal_time_constant_Foster=[7e-05, .0007, .01, .08] s  thermal_mass_initial_temperatures=[25, 25] degC  thermal_mass_initial_temperatures_Cauer=[25, 25, 25] degC  junction_thermal_mass=0.01 J/K  Tvec_initial_Foster=[25, 25, 25, 25] degC  no_thermal_network=0  junction_temperature_specify=off  junction_temperature_priority=None  junction_temperature=25 degC  junction_temperature_nominal_specify=off  junction_temperature_nominal_unit=degC  junction_temperature_nominal_value=1  Qj_specify=off  Qj_priority=None  Qj=0 W  Qj_nominal_specify=off  Qj_nominal_unit=W  Qj_nominal_value=1  accumulatedSwitchingLosses_specify=off  accumulatedSwitchingLosses_priority=None  accumulatedSwitchingLosses=0 J
  IGBT C(H) : ee_lib/Semiconductors & Converters/IGBT (Ideal, Switching)  port_option=ee.enum.controlport.ps  Vf=0.8 V  Ron=0.001 Ohm  Goff=1e-5 S  Vth=0.5 V  diode_param=2  diode_Vf=0.8 V  diode_Ron=0.001 Ohm  diode_Goff=1e-5 S  diode_C=5e-8 F  diode_iRM=-235 A  diode_iF=300 A  diode_idot=-50 A/us  diode_trr_param=1  diode_trr_factor=3  diode_trr=15 us  diode_Qrr=1.5e+3 s*uA  ice_specify=off  ice_priority=None  ice=0 A  ice_nominal_specify=off  ice_nominal_unit=A  ice_nominal_value=1  vce_specify=off  vce_priority=None  vce=0 V  vce_nominal_specify=off  vce_nominal_unit=V  vce_nominal_value=1  vge_specify=off  vge_priority=None  vge=0 V  vge_nominal_specify=off  vge_nominal_unit=V  vge_nominal_value=1  thermal_loss_option=ee.enum.converters.thermalLossOption.constantvalues  Von_data=[0, .1, .6, .8, 1, 1.3, 1.6, 2, 2.4; 0, .1, .7, 1, 1.2, 1.5, 1.9, 2.4, 2.8] V  Tj=[298.15, 398.15] K  Iout_data=[0, .1, 1, 5, 10, 20, 40, 70, 100] A  Eon_data=[0, .0024, .024, .12, .2, .48, 1.04, 2.16, 3.24; 0, .003, .03, .15, .25, .6, 1.3, 2.7, 4.05] * 1e-3 J  Eoff_data=[0, .0007, .0066, .033, .066, .17, .33, .83, 1.5; 0, .001, .01, .05, .1, .25, .5, 1.2, 2.2] * 1e-3 J  Eon_data_3D=[zeros(2, 9, 3)] J  Eoff_data_3D=[zeros(2, 9, 3)] J  Tj_loss=[298.15, 398.15] K  Iout_data_loss=[0, .1, 1, 5, 10, 20, 40, 70, 100] A  tabulateWithVce=false  Vce_loss=[0, 150, 300] V  Eon_scalar=22.86e-3 J  Eoff_scalar=17.14e-3 J  Voff=300 V  Iout_scalar=600 A  useCurrentFromPreviousCycle=false  useVoltageFromPreviousCycle=false  diodeModelType=ee.enum.converters.diodeModelType.pwl  diodeTableType=ee.enum.diode.tableType.IfMat  diode_IfMat=[.07, .12, .19, 1.75, 4.24, 7.32, 11.2; .16, .3, .72, 2.14, 4.02, 6.35, 9.12] A  diode_VfMat=[.9, 1.15, 1.25, 1.5, 1.75, 2.17, 2.6, 2.85; .58, .68, .75, 1.1, 1.38, 1.77, 2.27, 2.7] V  diode_TjVec=[25, 125] degC  diode_VfVec=[.5, .7, .9, 1.3, 1.7, 2.1, 2.5] V  diode_IfVec=[.1, .2, .5, 1, 2, 4, 7, 10] A  diode_Vr=-600 V  diode_Ls=150 nH  diode_Erec=0.03 J  diode_rec_loss_model=ee.enum.diode.reverseRecoveryModel.fixed  diode_ErecVal=0 J  diode_scaleWithIandV=true  diode_ErecMat=zeros(2, 3) J  diode_TjrecVec=[298.15, 398.15] K  diode_IfrecVec=[.1, 1, 10] A  diode_IrecVal=10 A  diode_VrecVal=10 V  diode_tFilter=1 / 1000 / 100 s  thermal_network_parameterization=ee.enum.thermalNetworkTopology.external  Rth=[.08, .5] K/W  Rth_Cauer=[.08, .1, .5] K/W  Rth_Foster=[.08, .14, .22, .16] K/W  thermal_mass_parameterization=ee.enum.thermalNetwork.timeconstant  thermal_mass=[.01, .5] J/K  thermal_mass_Cauer=[.01, .1, .5] J/K  thermal_mass_Foster=[.001, .005, .05, .5] J/K  thermal_time_constant=[.001, .2] s  thermal_time_constant_Cauer=[.001, .1, .2] s  thermal_time_constant_Foster=[7e-05, .0007, .01, .08] s  thermal_mass_initial_temperatures=[25, 25] degC  thermal_mass_initial_temperatures_Cauer=[25, 25, 25] degC  junction_thermal_mass=0.01 J/K  Tvec_initial_Foster=[25, 25, 25, 25] degC  no_thermal_network=0  junction_temperature_specify=off  junction_temperature_priority=None  junction_temperature=25 degC  junction_temperature_nominal_specify=off  junction_temperature_nominal_unit=degC  junction_temperature_nominal_value=1  Qj_specify=off  Qj_priority=None  Qj=0 W  Qj_nominal_specify=off  Qj_nominal_unit=W  Qj_nominal_value=1  accumulatedSwitchingLosses_specify=off  accumulatedSwitchingLosses_priority=None  accumulatedSwitchingLosses=0 J
  IGBT C(L) : ee_lib/Semiconductors & Converters/IGBT (Ideal, Switching)  port_option=ee.enum.controlport.ps  Vf=0.8 V  Ron=0.001 Ohm  Goff=1e-5 S  Vth=0.5 V  diode_param=2  diode_Vf=0.8 V  diode_Ron=0.001 Ohm  diode_Goff=1e-5 S  diode_C=5e-8 F  diode_iRM=-235 A  diode_iF=300 A  diode_idot=-50 A/us  diode_trr_param=1  diode_trr_factor=3  diode_trr=15 us  diode_Qrr=1.5e+3 s*uA  ice_specify=off  ice_priority=None  ice=0 A  ice_nominal_specify=off  ice_nominal_unit=A  ice_nominal_value=1  vce_specify=off  vce_priority=None  vce=0 V  vce_nominal_specify=off  vce_nominal_unit=V  vce_nominal_value=1  vge_specify=off  vge_priority=None  vge=0 V  vge_nominal_specify=off  vge_nominal_unit=V  vge_nominal_value=1  thermal_loss_option=ee.enum.converters.thermalLossOption.constantvalues  Von_data=[0, .1, .6, .8, 1, 1.3, 1.6, 2, 2.4; 0, .1, .7, 1, 1.2, 1.5, 1.9, 2.4, 2.8] V  Tj=[298.15, 398.15] K  Iout_data=[0, .1, 1, 5, 10, 20, 40, 70, 100] A  Eon_data=[0, .0024, .024, .12, .2, .48, 1.04, 2.16, 3.24; 0, .003, .03, .15, .25, .6, 1.3, 2.7, 4.05] * 1e-3 J  Eoff_data=[0, .0007, .0066, .033, .066, .17, .33, .83, 1.5; 0, .001, .01, .05, .1, .25, .5, 1.2, 2.2] * 1e-3 J  Eon_data_3D=[zeros(2, 9, 3)] J  Eoff_data_3D=[zeros(2, 9, 3)] J  Tj_loss=[298.15, 398.15] K  Iout_data_loss=[0, .1, 1, 5, 10, 20, 40, 70, 100] A  tabulateWithVce=false  Vce_loss=[0, 150, 300] V  Eon_scalar=22.86e-3 J  Eoff_scalar=17.14e-3 J  Voff=300 V  Iout_scalar=600 A  useCurrentFromPreviousCycle=false  useVoltageFromPreviousCycle=false  diodeModelType=ee.enum.converters.diodeModelType.pwl  diodeTableType=ee.enum.diode.tableType.IfMat  diode_IfMat=[.07, .12, .19, 1.75, 4.24, 7.32, 11.2; .16, .3, .72, 2.14, 4.02, 6.35, 9.12] A  diode_VfMat=[.9, 1.15, 1.25, 1.5, 1.75, 2.17, 2.6, 2.85; .58, .68, .75, 1.1, 1.38, 1.77, 2.27, 2.7] V  diode_TjVec=[25, 125] degC  diode_VfVec=[.5, .7, .9, 1.3, 1.7, 2.1, 2.5] V  diode_IfVec=[.1, .2, .5, 1, 2, 4, 7, 10] A  diode_Vr=-600 V  diode_Ls=150 nH  diode_Erec=0.03 J  diode_rec_loss_model=ee.enum.diode.reverseRecoveryModel.fixed  diode_ErecVal=0 J  diode_scaleWithIandV=true  diode_ErecMat=zeros(2, 3) J  diode_TjrecVec=[298.15, 398.15] K  diode_IfrecVec=[.1, 1, 10] A  diode_IrecVal=10 A  diode_VrecVal=10 V  diode_tFilter=1 / 1000 / 100 s  thermal_network_parameterization=ee.enum.thermalNetworkTopology.external  Rth=[.08, .5] K/W  Rth_Cauer=[.08, .1, .5] K/W  Rth_Foster=[.08, .14, .22, .16] K/W  thermal_mass_parameterization=ee.enum.thermalNetwork.timeconstant  thermal_mass=[.01, .5] J/K  thermal_mass_Cauer=[.01, .1, .5] J/K  thermal_mass_Foster=[.001, .005, .05, .5] J/K  thermal_time_constant=[.001, .2] s  thermal_time_constant_Cauer=[.001, .1, .2] s  thermal_time_constant_Foster=[7e-05, .0007, .01, .08] s  thermal_mass_initial_temperatures=[25, 25] degC  thermal_mass_initial_temperatures_Cauer=[25, 25, 25] degC  junction_thermal_mass=0.01 J/K  Tvec_initial_Foster=[25, 25, 25, 25] degC  no_thermal_network=0  junction_temperature_specify=off  junction_temperature_priority=None  junction_temperature=25 degC  junction_temperature_nominal_specify=off  junction_temperature_nominal_unit=degC  junction_temperature_nominal_value=1  Qj_specify=off  Qj_priority=None  Qj=0 W  Qj_nominal_specify=off  Qj_nominal_unit=W  Qj_nominal_value=1  accumulatedSwitchingLosses_specify=off  accumulatedSwitchingLosses_priority=None  accumulatedSwitchingLosses=0 J
  Mux : Mux  Inputs=3
  PS-Simulink Converter : nesl_utility/PS-Simulink Converter  PhysicalDomain=network_engine_domain  SubClassName=ps_output  LeftPortType=input  RightPortType=output  PseudoPeriodic=off  Frequencies=[]  VectorFormat=inherit  Unit=inherit  AffineConversion=off
  PS-Simulink Converter1 : nesl_utility/PS-Simulink Converter  PhysicalDomain=network_engine_domain  SubClassName=ps_output  LeftPortType=input  RightPortType=output  PseudoPeriodic=off  Frequencies=[]  VectorFormat=inherit  Unit=inherit  AffineConversion=off
  PS-Simulink Converter2 : nesl_utility/PS-Simulink Converter  PhysicalDomain=network_engine_domain  SubClassName=ps_output  LeftPortType=input  RightPortType=output  PseudoPeriodic=off  Frequencies=[]  VectorFormat=inherit  Unit=inherit  AffineConversion=off
  Phase Splitter : ee_lib/Connectors & References/Phase Splitter
  Simulink-PS G{1..6} (6 alike) : nesl_utility/Simulink-PS Converter  PhysicalDomain=network_engine_domain  SubClassName=ps_input  LeftPortType=input  RightPortType=output  PseudoPeriodic=off  Frequencies=[]  NoiseDistribution=none  NoiseParameters=[]  Unit=1  AffineConversion=off  FilteringAndDerivatives=zero  SimscapeFilterOrder=1  InputFilterTimeConstant=1e-6  UdotUserProvided=0
  Voltage Sensor : fl_lib/Electrical/Electrical Sensors/Voltage Sensor
  Voltage Sensor1 : fl_lib/Electrical/Electrical Sensors/Voltage Sensor
  Voltage Sensor2 : fl_lib/Electrical/Electrical Sensors/Voltage Sensor
  Connection Port : PMIOPort  Side=Right
  + : PMIOPort  Port=2  Side=Left
  - : PMIOPort  Port=3  Side=Left
  Vabc : Outport
  wires:
  GatePulses/1 -> Demux/1
  Demux/1 -> Simulink-PS G1/1  "G_AH"
  Demux/2 -> Simulink-PS G2/1  "G_AL"
  Demux/3 -> Simulink-PS G3/1  "G_BH"
  Demux/4 -> Simulink-PS G4/1  "G_BL"
  Demux/5 -> Simulink-PS G5/1  "G_CH"
  Demux/6 -> Simulink-PS G6/1  "G_CL"
  PS-Simulink Converter/1 -> Mux/1  "Va"
  PS-Simulink Converter1/1 -> Mux/2  "Vb"
  PS-Simulink Converter2/1 -> Mux/3  "Vc"
  Mux/1 -> Vabc/1
  connections:
  Connection Port/RConn1 -- Phase Splitter/LConn1
  Simulink-PS G1/RConn1 -- IGBT A(H)/LConn1
  Simulink-PS G2/RConn1 -- IGBT A(L)/LConn1
  Simulink-PS G3/RConn1 -- IGBT B(H)/LConn1
  Simulink-PS G4/RConn1 -- IGBT B(L)/LConn1
  IGBT A(H)/RConn2 -- Voltage Sensor/LConn1 -- Phase Splitter/RConn1 -- IGBT A(L)/RConn1
  IGBT B(H)/RConn2 -- Voltage Sensor1/LConn1 -- Phase Splitter/RConn2 -- IGBT B(L)/RConn1
  IGBT C(H)/RConn2 -- Voltage Sensor2/LConn1 -- Phase Splitter/RConn3 -- IGBT C(L)/RConn1
  Simulink-PS G5/RConn1 -- IGBT C(H)/LConn1
  Simulink-PS G6/RConn1 -- IGBT C(L)/LConn1
  +/RConn1 -- IGBT C(H)/RConn1 -- IGBT B(H)/RConn1 -- IGBT A(H)/RConn1
  -/RConn1 -- Voltage Sensor2/RConn2 -- IGBT C(L)/RConn2 -- Voltage Sensor1/RConn2 -- IGBT B(L)/RConn2 -- Voltage Sensor/RConn2 -- IGBT A(L)/RConn2
  PS-Simulink Converter/LConn1 -- Voltage Sensor/RConn1
  PS-Simulink Converter1/LConn1 -- Voltage Sensor1/RConn1
  PS-Simulink Converter2/LConn1 -- Voltage Sensor2/RConn1

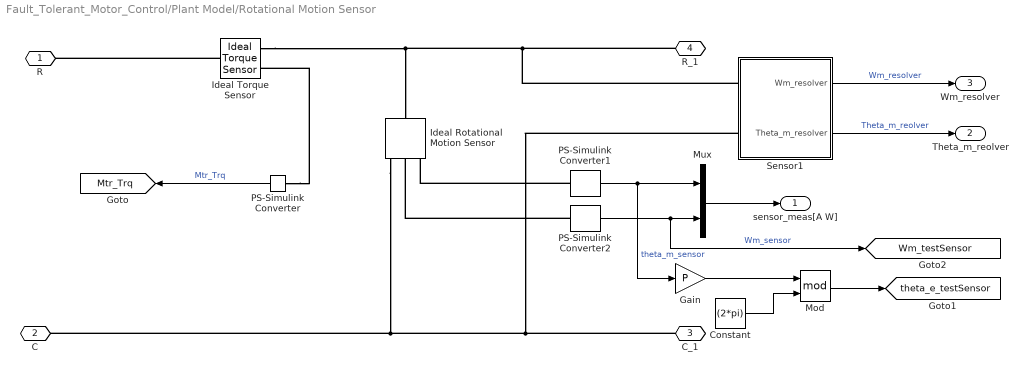
== system Fault_Tolerant_Motor_Control/Plant Model/Rotational Motion Sensor ==
  Constant : Constant  Value=(2*pi)
  Gain : Gain  Gain=P
  Ideal Rotational Motion Sensor : fl_lib/Mechanical/Mechanical Sensors/Ideal Rotational Motion Sensor  reference=foundation.enum.MeasurementReference.difference  acceleration_port=false  velocity_port=true  position_port=true  wrap_angle=true  offset=0 rad
  Ideal Torque Sensor : fl_lib/Mechanical/Mechanical Sensors/Ideal Torque Sensor
  Mod : Math  Operator=mod
  Mux : Mux  Inputs=2
  PS-Simulink Converter : nesl_utility/PS-Simulink Converter  PhysicalDomain=network_engine_domain  SubClassName=ps_output  LeftPortType=input  RightPortType=output  PseudoPeriodic=off  Frequencies=[]  VectorFormat=inherit  Unit=inherit  AffineConversion=off
  PS-Simulink Converter1 : nesl_utility/PS-Simulink Converter  PhysicalDomain=network_engine_domain  SubClassName=ps_output  LeftPortType=input  RightPortType=output  PseudoPeriodic=off  Frequencies=[]  VectorFormat=1-D array  Unit=rad  AffineConversion=off
  PS-Simulink Converter2 : nesl_utility/PS-Simulink Converter  PhysicalDomain=network_engine_domain  SubClassName=ps_output  LeftPortType=input  RightPortType=output  PseudoPeriodic=off  Frequencies=[]  VectorFormat=1-D array  Unit=rad/s  AffineConversion=off
  Sensor1 : Subsystem
  R : PMIOPort  Side=Left
  C : PMIOPort  Port=2  Side=Left
  C_1 : PMIOPort  Port=3  Side=Right
  R_1 : PMIOPort  Port=4  Side=Right
  sensor_meas[A W] : Outport
  Theta_m_reolver : Outport  Port=2
  Wm_resolver : Outport  Port=3
  tag scope: Mtr_Trq=global, Wm_testSensor=global, theta_e_testSensor=global
  wires:
  PS-Simulink Converter/1 -> [Mtr_Trq]  "Mtr_Trq"
  PS-Simulink Converter1/1 -> Gain/1, Mux/1  "theta_m_sensor"
  PS-Simulink Converter2/1 -> [Wm_testSensor], Mux/2  "Wm_sensor"
  Mux/1 -> sensor_meas[A W]/1
  Sensor1/1(Wm_resolver) -> Wm_resolver/1  "Wm_resolver"
  Sensor1/2(Theta_m_resolver) -> Theta_m_reolver/1  "Theta_m_reolver"
  Gain/1 -> Mod/1
  Constant/1 -> Mod/2
  Mod/1 -> [theta_e_testSensor]
  connections:
  C_1/RConn1 -- Ideal Rotational Motion Sensor/RConn1 -- C/RConn1 -- Sensor1/LConn2
  Ideal Torque Sensor/LConn1 -- R/RConn1
  Ideal Torque Sensor/RConn1 -- Sensor1/LConn1 -- R_1/RConn1 -- Ideal Rotational Motion Sensor/LConn1
  PS-Simulink Converter/LConn1 -- Ideal Torque Sensor/RConn2
  PS-Simulink Converter1/LConn1 -- Ideal Rotational Motion Sensor/RConn3
  PS-Simulink Converter2/LConn1 -- Ideal Rotational Motion Sensor/RConn2

== system Fault_Tolerant_Motor_Control/Controller/Field Oriented Control/Inner Loop Controller ==
  Idq_ref : Inport
  W_e : Inport  Port=2
  Iabc : Inport  Port=3
  Theta_e : Inport  Port=4
  Bias : Bias  Bias=theta_offset  SaturateOnIntegerOverflow=off
  Constant : Constant  Value=0  SampleTime=-1
  Constant1 : Constant  Value=Vdc
  Gain : Gain  Gain=1/sqrt(3)
  PMSM Current Controller with Pre Control : eePmsmCurrentController/PMSM Current Controller with Pre-Control  Kp_id=Kp_Id  Ki_id=Ki_Iq  Kaw_id=800  Kp_iq=Kp_Iq  Ki_iq=Ki_Iq  Kaw_iq=800  Ts=Ts  Tsd=0.001  AxisPrio=Q-axis  ActZC=off  ActFF=on  idVect=[-Imax,Imax]  iqVect=[-Imax,Imax]  LdMatrix=[Ld,Ld;Ld,Ld]  LqMatrix=[Lq,Lq;Lq,Lq]  psimMatrix=[Psi,Psi;Psi,Psi]
      settings: LibrarySourceBlock=|
      | eePmsmFieldOrientedControl/PMSM Field-Oriented
      | Control/Inner loop control/PMSM Current Controller
      | with Pre-Control
  Park Transform : eeTransforms/Park Transform  AxisAlignment=Q-axis  PowerInvariant=off
      settings: LibrarySourceBlock=|
      | eePmsmFieldOrientedControl/PMSM Field-Oriented
      | Control/Inner loop control/Park Transform
  Selector : Selector  InputPortWidth=3  IndexOptions=Index vector (dialog)  Indices=[1 2]  OutputSizes=1
  Vdq_Ref : Outport  VectorParamsAs1DForOutWhenUnconnected=off
  Idq : Outport  Port=2  VectorParamsAs1DForOutWhenUnconnected=off
  wires:
  Bias/1 -> Park Transform/2
  Gain/1 -> PMSM Current Controller with Pre Control/4
  Park Transform/1 -> Selector/1
  Iabc/1 -> Park Transform/1
  Constant/1 -> PMSM Current Controller with Pre Control/5
  Idq_ref/1 -> PMSM Current Controller with Pre Control/1
  Theta_e/1 -> Bias/1
  Selector/1 -> Idq/1, PMSM Current Controller with Pre Control/2
  W_e/1 -> PMSM Current Controller with Pre Control/3
  PMSM Current Controller with Pre Control/1 -> Vdq_Ref/1
  Constant1/1 -> Gain/1

== system Fault_Tolerant_Motor_Control/Controller/Field Oriented Control/Outer Loop Control ==
  Wm_ref : Inport
  Wm : Inport  Port=2
  Constant : Constant  Value=0
  Constant1 : Constant  Value=Vdc
  Current Refrence Generation : Subsystem
  Torque Controller : Subsystem
  Idq_ref : Outport
  wires:
  Wm_ref/1 -> Torque Controller/1(wRef)
  Torque Controller/1(TqRefUnsat) -> Current Refrence Generation/1(TqRef)
  Current Refrence Generation/1(TqRefSat) -> Torque Controller/3(TqRefSat)
  Wm/1 -> Current Refrence Generation/2(wMechanical), Torque Controller/2(wMechanical)
  Constant/1 -> Torque Controller/4(Reset)
  Current Refrence Generation/2(Idq_ref) -> Idq_ref/1
  Constant1/1 -> Current Refrence Generation/3(Vdc)

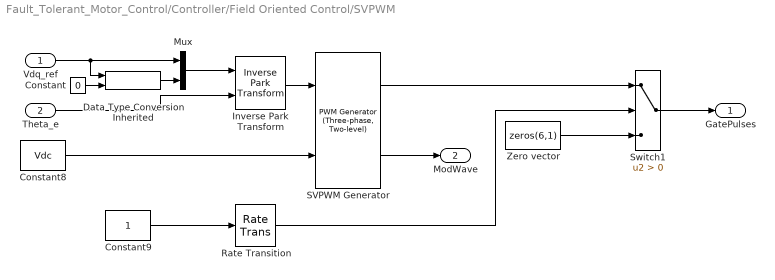
== system Fault_Tolerant_Motor_Control/Controller/Field Oriented Control/SVPWM ==
  Vdq_ref : Inport
  Theta_e : Inport  Port=2
  Constant : Constant  Value=0  SampleTime=Tsc
  Constant8 : Constant  Value=Vdc
  Constant9 : Constant
  Data Type Conversion Inherited : simulink/Signal Attributes/Data Type Conversion Inherited  ConvertRealWorld=Real World Value  DoSatur=off
  Inverse Park Transform : eeTransforms/Inverse Park Transform  AxisAlignment=Q-axis  PowerInvariant=off
      settings: LibrarySourceBlock=|
      | eePmsmFieldOrientedControl/PMSM Field-Oriented
      | Control/PWM/Inverse
      | Park Transform
  Mux : Mux  Inputs=2
  Rate Transition : RateTransition  OutPortSampleTime=Ts
  SVPWM Generator : eePwmGeneratorTwoLevel/PWM Generator (Three-phase, Two-level)  PWMMode=Continuous PWM (CPWM)  CPWMMode=SVM: space vector modulation  DPWMMode=60 DPWM: 60 degree discontinuous PWM  fsw=Fsw  Ts=Ts
      settings: LibrarySourceBlock=|
      | eePmsmFieldOrientedControl/PMSM Field-Oriented
      | Control/PWM/PWM Generator
      | (Three-phase, Two-level)
  Switch1 : Switch  Criteria=u2 > Threshold  SaturateOnIntegerOverflow=off  InputSameDT=off
  Zero vector : Constant  Value=zeros(6,1)  SampleTime=Ts
  GatePulses : Outport  VectorParamsAs1DForOutWhenUnconnected=off
  ModWave : Outport  Port=2  SampleTime=Tsc  VectorParamsAs1DForOutWhenUnconnected=off
  wires:
  Mux/1 -> Inverse Park Transform/1
  Data Type Conversion Inherited/1 -> Mux/2
  SVPWM Generator/1 -> Switch1/1
  Zero vector/1 -> Switch1/3
  SVPWM Generator/2 -> ModWave/1
  Vdq_ref/1 -> Data Type Conversion Inherited/1, Mux/1
  Constant/1 -> Data Type Conversion Inherited/2
  Rate Transition/1 -> Switch1/2
  Theta_e/1 -> Inverse Park Transform/2
  Switch1/1 -> GatePulses/1
  Inverse Park Transform/1 -> SVPWM Generator/1
  Constant8/1 -> SVPWM Generator/2
  Constant9/1 -> Rate Transition/1
